simulink model "mehrw5"  (Simulink 4.00)
settings: Solver=ode45  SolverMode=SingleTasking  StartTime=0.0  StopTime=30  FixedStep=0.1  MaxStep=0.1  RelTol=1e-3  AbsTol=1e-6
values from neighbouring files (symbols this model uses):
  a = -1    [fmasse_var_1.m]    (also in fmasse_var_2.m; mehrw_4.m = my_system1.a; mehrw_5.m = my_system1.a)
  b = 1    [anw_pid_1.m]    (also in mehrw_4.m = my_system1.b; mehrw_5.m = my_system1.b)
  Cy = zeros(1,10);				Cy(1,10) = 1    [mehrw_1.m]    (also in mehrw_2.m; mehrw_3.m; mehrw_4.m; mehrw_5.m)
  rT = 0.1    [mehrw_1.m]    (also in mehrw_2.m; mehrw_3.m; mehrw_4.m; mehrw_5.m)
  Ts = 0.5    [mehrw_4.m]    (also in mehrw_5.m; pbeisp_5.m = 0.1)
settings Model: LastModifiedBy=Administrator  Refine=3  SaveTime=off  SaveOutput=off  LimitDataPoints=off  BlockReductionOpt=off

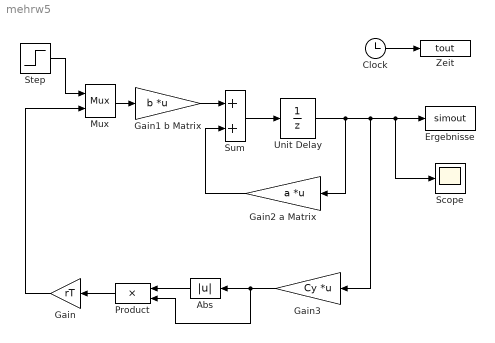
== system mehrw5 ==
  Abs : Abs  Orientation=left  SaturateOnIntegerOverflow=on
  Clock : Clock
      settings: DisplayTime=off  Decimation=10
  Ergebnisse : ToWorkspace  VariableName=simout  SampleTime=0  SaveFormat=Array
      settings: MaxDataPoints=1000
  Gain : Gain  Orientation=left  Gain=rT  Multiplication=Element-wise(K.*u)  SaturateOnIntegerOverflow=on
  Gain1 b Matrix : Gain  Gain=b  Multiplication=Matrix(K*u)  SaturateOnIntegerOverflow=on
  Gain2 a Matrix : Gain  Orientation=left  Gain=a  Multiplication=Matrix(K*u)  SaturateOnIntegerOverflow=on
  Gain3 : Gain  Orientation=left  Gain=Cy  Multiplication=Matrix(K*u)  SaturateOnIntegerOverflow=on
  Mux : Mux  Inputs=2
      settings: DisplayOption=none
  Product : Product  Orientation=left  Inputs=2  Multiplication=Element-wise(.*)  SaturateOnIntegerOverflow=on
  Scope : Scope
      settings: TickLabels=on  TimeRange=30  YMin=-41.6038  YMax=41.6038  SaveToWorkspace=off  SaveName=ScopeData  DataFormat=Array  LimitDataPoints=on  MaxDataPoints=5000
  Step : Step  Time=0  Before=0  After=1  SampleTime=Ts
  Sum : Sum  Inputs=++  SaturateOnIntegerOverflow=on
  Unit Delay : UnitDelay  X0=0  SampleTime=Ts
  Zeit : ToWorkspace  VariableName=tout  SampleTime=0  SaveFormat=Array
      settings: MaxDataPoints=1000
  wires:
  Gain3/1 -> Product/2, Abs/1
  Product/1 -> Gain/1
  Gain/1 -> Mux/2
  Abs/1 -> Product/1
  Step/1 -> Mux/1
  Mux/1 -> Gain1 b Matrix/1
  Clock/1 -> Zeit/1
  Unit Delay/1 -> Gain2 a Matrix/1, Ergebnisse/1, Scope/1, Gain3/1
  Gain1 b Matrix/1 -> Sum/1
  Sum/1 -> Unit Delay/1
  Gain2 a Matrix/1 -> Sum/2
